simulink model "My_Linear_new"  (R2021b)
settings: Solver=VariableStepAuto  StartTime=0.0  StopTime=simTime  RelTol=1e-3
values from neighbouring files (symbols this model uses):
  Aa = [0 0 0 0 0 0 0 0 0 0 0 0 ... (144 elements, 12x12)]    [Linear_System_parameters.mat]
  Bb = [0 0 0 0 0 0.442944691806 0 0 0 16610.4259426 0 22147.2345902 ... (48 elements, 12x4)]    [Linear_System_parameters.mat]
  Cc = [1 0 0 0 0 0 0 1 0 0 0 0 ... (72 elements, 6x12)]    [Linear_System_parameters.mat]
  Dd = [0 0 0 0 0 0 0 0 0 0 0 0 ... (24 elements, 6x4)]    [Linear_System_parameters.mat]
  uss = [11.0736172952 11.0736172952 11.0736172952 11.0736172952]    [Linear_System_parameters.mat]
  xss = [9.13004546083e-32 -1.57965453512e-31 -3.8506255354e-32 -6.4400908867e-27 6.81940918243e-28 1.19743344099e-15 0 0 0 -1.28453386059e-24 3.4686873125e-26 -3.08292593178e-24]    [Linear_System_parameters.mat]
undefined symbols (not defined in the file or in its folder): RPM, TakeStep, x0
settings Model: Creator=tanzc  LastModifiedBy=tanzc

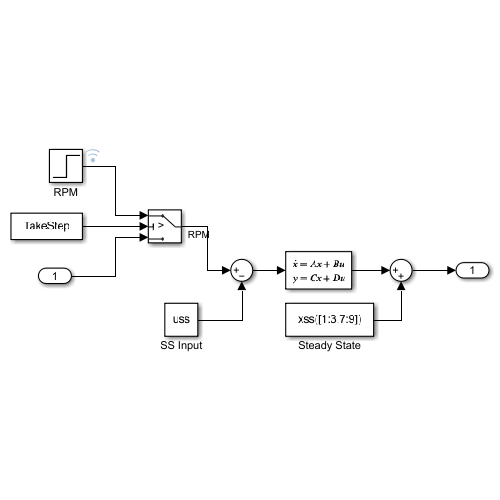
[thumbnail: Simulink's stored preview of the top-level diagram]
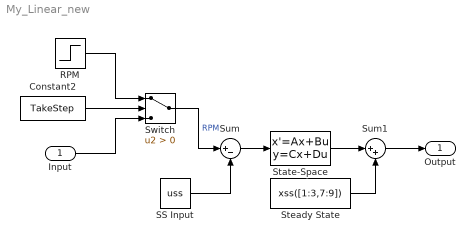
== system My_Linear_new ==
  Input : Inport
  Constant2 : Constant  Value=TakeStep
  RPM : Step  Time=0  After=RPM  SampleTime=0
  SS Input : Constant  Value=uss  VectorParams1D=off
  State-Space : StateSpace  A=Aa  B=Bb  C=Cc  D=Dd  InitialCondition=x0
  Steady State : Constant  Value=xss([1:3,7:9])  VectorParams1D=off
  Sum : Sum  Inputs=|+-
  Sum1 : Sum  Inputs=|++
  Switch : Switch  Criteria=u2 > Threshold
  Output : Outport
  wires:
  Switch/1 -> Sum/1  "RPM"
  Constant2/1 -> Switch/2
  RPM/1 -> Switch/1
  Sum/1 -> State-Space/1
  Sum1/1 -> Output/1
  SS Input/1 -> Sum/2
  Input/1 -> Switch/3
  Steady State/1 -> Sum1/2
  State-Space/1 -> Sum1/1
